simulink model "Copy_of_LTI"  (Simulink 8.0)
settings: Solver=ode45  StartTime=0.0  StopTime=10.0  RelTol=1e-3
undefined symbols (not defined in the file): A, B, C, D, var, x0
settings Model: Creator=chepeadan  LastModifiedBy=koehler
settings DataIOCC: SignalLoggingSaveFormat=ModelDataLogs
settings DebuggingCC: FcnCallInpInsideContextMsg=UseLocalSettings  StrictBusMsg=Warning
settings GRTTargetCC: CombineOutputUpdateFcns=off  GRTInterface=on

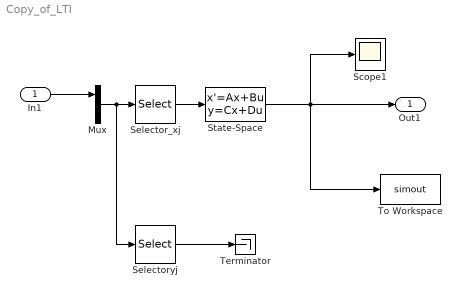
== system Copy_of_LTI ==
  In1 : Inport
  Mux : Mux  Inputs=2
  Scope1 : Scope
      settings: TimeRange=0.5847953216374258  YMin=-0.1657458563535892  YMax=1.21546961325967
  Selector_xj : Selector  InputPortWidth=2  IndexOptions=Index vector (dialog)  Indices=[1]  OutputSizes=1
  Selectoryj : Selector  InputPortWidth=2  IndexOptions=Index vector (dialog)  Indices=[2]  OutputSizes=1
  State-Space : StateSpace  A=A  B=B  C=C  D=D  X0=x0+var*rand(1)
  Terminator : Terminator
  To Workspace : ToWorkspace  VariableName=simout  SampleTime=-1  SaveFormat=Structure With Time
  Out1 : Outport
  wires:
  In1/1 -> Mux/1
  State-Space/1 -> Out1/1, To Workspace/1, Scope1/1
  Mux/1 -> Selectoryj/1, Selector_xj/1
  Selector_xj/1 -> State-Space/1
  Selectoryj/1 -> Terminator/1
